simulink model "NL_PID"  (R2015a)
settings: Solver=ode45  StartTime=0.0  StopTime=10.0  RelTol=1e-3
undefined symbols (not defined in the file or in its folder): Cn, J2, Kc, Ke, Kg, Kr, Ks, L, mu, n, p, R, Rchn, rCn, rRch, tau_d, tau_i
settings Model: Creator=m2istr_13  LastModifiedBy=David
settings OptimizationCC: ExpressionDepthLimit=2147483647
settings DebuggingCC: UnderspecifiedInitializationDetection=Classic  MergeDetectMultiDrivingBlocksExec=none  SolverPrmCheckMsg=warning  StateNameClashWarn=warning

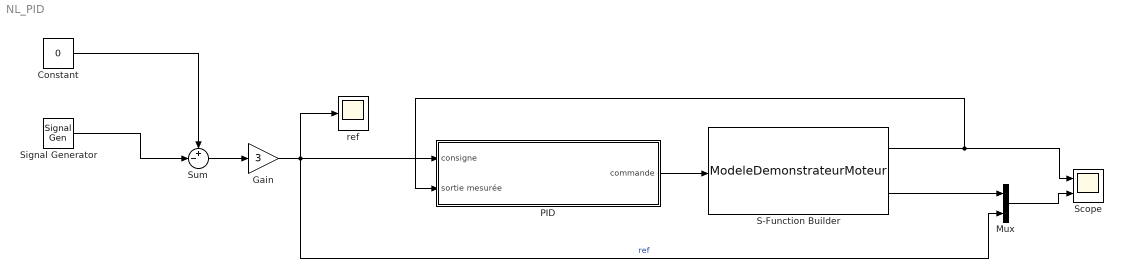
== system NL_PID ==
  Constant : Constant  Value=0
  Gain : Gain  Gain=3
  Mux : Mux  Inputs=2
  PID : Subsystem
  S-Function Builder : S-Function  InitFcn=try, set_param(gcb,'FunctionName','ModeleDemonstrateurMoteur'), end  FunctionName=ModeleDemonstrateurMoteur  Parameters=R,L,Ke,Kc,mu,J2,Cn,rCn,2*rand(1)-1,Ks,Kr,Kg,0.01,Rchn,rRch,2*rand(1)-1  SFunctionModules=ModeleDemonstrateurMoteur_wrapper  mask(S-Function Builder){}
      mask help: Simulink:masks:SFunctionBuilder_MD
      mask init:
      | val = [[.9  0.75 0.75 1 1 .9 .9 1]',[1 1 0.75 0.75 .9 .9 1 .9]'];try , sys = get_param(gcb,'SfunBuilderFcnName');if isempty(sys), sys = get_param(gcb,'FunctionName'); end,catch, sys = get_param(gcb,'FunctionName'); end
      settings: CopyFcn=set_param(gcbh,'LinkStatus','none')  PreSaveFcn=try, set_param(gcb,'FunctionName','ModeleDemonstrateurMoteur'), end  OpenFcn=sfunctionwizard(gcbh)
      mask Display: plot(val(:,1),val(:,2)),disp(sys), port_label('input',1,'Vm'), port_label('output',1,'Vs'), port_label('output',2,'Vg')
  Scope : Scope  NumInputPorts=2
      settings: YMin=-5~2.9  YMax=5~4.9  SaveName=ScopeData4
  Signal Generator : SignalGenerator  WaveForm=square  Frequency=0.2
  Sum : Sum  Inputs=+-|
  ref : Scope
      settings: SaveName=ScopeData3
  wires:
  Signal Generator/1 -> Sum/2
  Constant/1 -> Sum/1
  Sum/1 -> Gain/1
  Gain/1 -> Mux/2, PID/1(consigne), ref/1  "ref"
  Mux/1 -> Scope/2
  S-Function Builder/1 -> PID/2(sortie mesurée), Scope/1
  S-Function Builder/2 -> Mux/1
  PID/1(commande) -> S-Function Builder/1

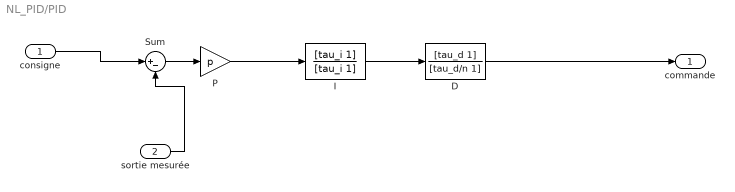
== system NL_PID/PID ==
  consigne : Inport
  sortie mesurée : Inport  Port=2
  D : TransferFcn  Numerator=[tau_d 1]  Denominator=[tau_d/n 1]
  I : TransferFcn  Numerator=[tau_i 1]  Denominator=[tau_i 1]
  P : Gain  Gain=p
  Sum : Sum  Inputs=|+-
  commande : Outport
  wires:
  I/1 -> D/1
  D/1 -> commande/1
  P/1 -> I/1
  Sum/1 -> P/1
  sortie mesurée/1 -> Sum/2
  consigne/1 -> Sum/1
